simulink model "gm_sampleModel1902_1_sub"  (R2023a)
settings: Solver=VariableStepAuto  StartTime=0.0  StopTime=10.0  RelTol=1e-3
libraries: hdlsllib x2, simulink x1
settings Model: Creator=user1  LastModifiedBy=user1
settings OptimizationCC: BlockReduction=off  ConditionallyExecuteInputs=off
settings DebuggingCC: InheritedTsInSrcMsg=none

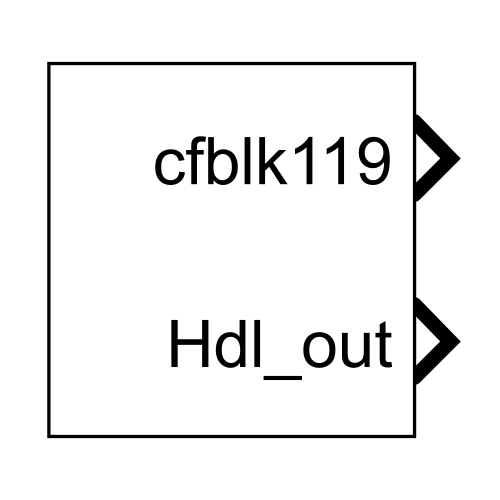
[thumbnail: Simulink's stored preview of the top-level diagram]
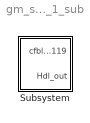
== system gm_sampleModel1902_1_sub ==
  Subsystem : Subsystem

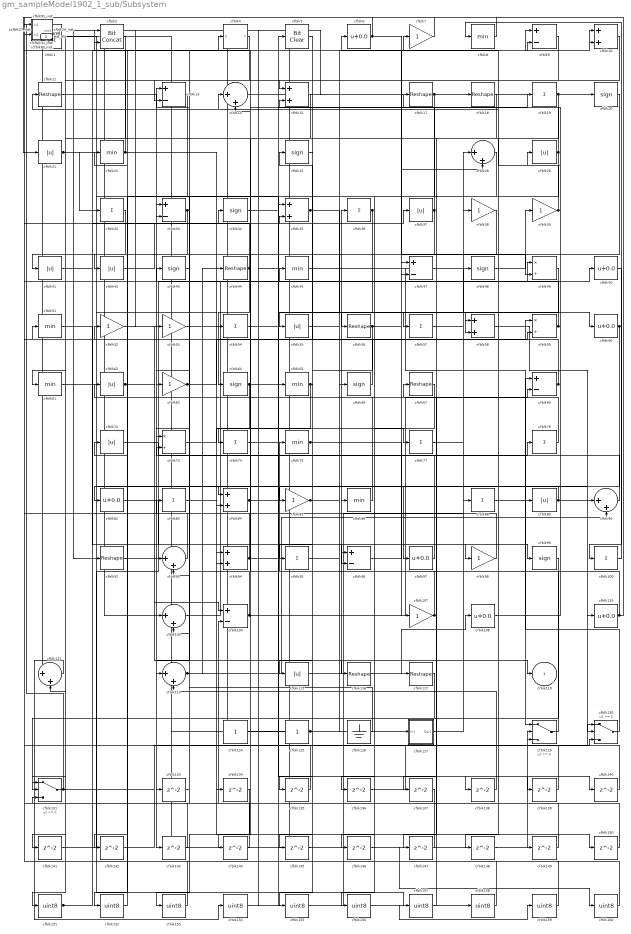
== system gm_sampleModel1902_1_sub/Subsystem ==
  cfblk1 : hdlsllib/Logic and Bit Operations/Interval Test  IntervalClosedRight=on  uplimit=0.5  IntervalClosedLeft=on  lowlimit=-0.5  OutDataTypeStr=uint8
  cfblk{10,15,35,58,84,94} (6 alike) : Sum  OutDataTypeStr=uint8
  cfblk{19,32,36,54,57,74,77,79,83,88,95,100} (12 alike) : Sum  Inputs=+  OutDataTypeStr=uint8
  cfblk{14,28,90,93,103,111,113} (7 alike) : Sum  Inputs=|++  OutDataTypeStr=uint8
  cfblk{9,13,33,47,69,96,104} (7 alike) : Sum  Inputs=+-  OutDataTypeStr=uint8
  cfblk105_inst : Subsystem
  cfblk{7,38..39,52..53,63,85,98,107} (9 alike) : Gain  OutDataTypeStr=uint8
  cfblk{6,50,60,82,97,108,110} (7 alike) : Bias  Bias=0.0  SaturateOnIntegerOverflow=off
  cfblk109_inst : Subsystem
  cfblk{11,17..18,44,56,67,92,116..117} (9 alike) : Reshape
  cfblk112_inst : Subsystem
  cfblk{21,29,37,41..42,55,62,72,89,115} (10 alike) : Abs  OutDataTypeStr=uint8  SaturateOnIntegerOverflow=off
  cfblk124 : Constant  OutDataTypeStr=uint8  SampleTime=-1
  cfblk125 : Constant  OutDataTypeStr=uint8  SampleTime=-1
  cfblk126 : Ground
  cfblk127 : Subsystem
  cfblk129 : Switch  OutDataTypeStr=uint8  SaturateOnIntegerOverflow=off  InputSameDT=off
  cfblk130 : Switch  OutDataTypeStr=uint8  SaturateOnIntegerOverflow=off  InputSameDT=off
  cfblk131 : Switch  OutDataTypeStr=uint8  SaturateOnIntegerOverflow=off  InputSameDT=off
  cfblk{133..150} (18 alike) : Delay  SampleTime=1
  cfblk{151..160} (10 alike) : DataTypeConversion  OutDataTypeStr=uint8  SaturateOnIntegerOverflow=off  RndMeth=Floor
  cfblk2 : hdlsllib/Logic and Bit Operations/Bit Concat  numInputs=2
  cfblk{20,25,34,43,48,64,66,99} (8 alike) : Signum
  cfblk{8,22,45,51,61,65,75,86} (8 alike) : MinMax  OutDataTypeStr=uint8
  cfblk24_inst : Subsystem
  cfblk26_inst : Subsystem
  cfblk27_inst : Subsystem
  cfblk31_inst : Subsystem
  cfblk4 : Subsystem  mask(Detect Rise Nonnegative){vinit=double(0), InputProcessing=Elements as channels (sample based), OutDataTypeStr=uint8}
      mask prompts: vinit "Simulink:masks:InitialCondition_MP"; InputProcessing "Simulink:masks:InputProcessing_MP"; OutDataTypeStr "Simulink:masks:OutputDataType_MP"
      mask help: Simulink:masks:DetectRiseNonnegative_MD
      mask init:
      | InputProcessing = 'Elements as channels (sample based)';
      | OutDataTypeStr = 'uint8';
      | vinit = double(0);
      mask TypeOptions InputProcessing: Simulink:masks:ColumnsAsChannelsFrameBased | Simulink:masks:ElementsAsChannelsSampleBased
      mask TypeOptions OutDataTypeStr: Simulink:masks:uint8 | Simulink:masks:boolean
      mask Display: fprintf('U >= 0\n&  NOT\nU/z >= 0')
  cfblk49 : Product  Inputs=*/  OutDataTypeStr=uint8  RndMeth=Zero  SaturateOnIntegerOverflow=on
  cfblk5 : simulink/Logic and Bit Operations/Bit Clear  iBit=0
      settings: LibrarySourceBlock=|
      | hdlsllib/Logic and Bit
      | Operations/Bit Clear
  cfblk59 : Product  Inputs=*/  OutDataTypeStr=uint8  RndMeth=Zero  SaturateOnIntegerOverflow=on
  cfblk73 : Product  Inputs=*/  OutDataTypeStr=uint8  RndMeth=Zero  SaturateOnIntegerOverflow=on
  cfblk80_inst : Subsystem
  cfblk91_inst : Subsystem
  cfblk119 : Outport  OutDataTypeStr=uint8  SampleTime=1  VectorParamsAs1DForOutWhenUnconnected=off
  Hdl_out : Outport  Port=2  OutDataTypeStr=uint8  SampleTime=1
  wires:
  cfblk1/1 -> cfblk157/1, cfblk111/2
  cfblk10/1 -> cfblk15/1
  cfblk100/1 -> cfblk8/1
  cfblk103/1 -> cfblk45/1
  cfblk104/1 -> cfblk69/2, cfblk112_inst/1(in1)
  cfblk105_inst/1(out1) -> cfblk127/1(In1)
  cfblk107/1 -> cfblk147/1, cfblk36/1
  cfblk108/1 -> cfblk15/2
  cfblk109_inst/1(out1) -> cfblk117/1
  cfblk11/1 -> cfblk143/1
  cfblk110/1 -> cfblk21/1, cfblk75/1
  cfblk111/1 -> cfblk154/1
  cfblk112_inst/1(out1) -> cfblk92/1
  cfblk113/1 -> cfblk90/2, cfblk44/1
  cfblk115/1 -> cfblk86/1
  cfblk116/1 -> cfblk108/1
  cfblk117/1 -> cfblk133/1
  cfblk124/1 -> cfblk35/1
  cfblk125/1 -> cfblk66/1, Hdl_out/1
  cfblk126/1 -> cfblk51/1
  cfblk127/1(Out1) -> cfblk88/1
  cfblk129/1 -> cfblk4/1(U)
  cfblk13/1 -> cfblk152/1
  cfblk130/1 -> cfblk69/1
  cfblk131/1 -> cfblk130/3, cfblk109_inst/2(in2)
  cfblk133/1 -> cfblk103/2
  cfblk134/1 -> cfblk153/1
  cfblk135/1 -> cfblk93/2
  cfblk136/1 -> cfblk130/1
  cfblk137/1 -> cfblk131/3
  cfblk138/1 -> cfblk113/2
  cfblk139/1 -> cfblk91_inst/2(in2)
  cfblk14/1 -> cfblk10/1
  cfblk140/1 -> cfblk105_inst/1(in1)
  cfblk141/1 -> cfblk49/1
  cfblk142/1 -> cfblk129/2
  cfblk143/1 -> cfblk112_inst/2(in2)
  cfblk144/1 -> cfblk27_inst/2(in2)
  cfblk145/1 -> cfblk1/1
  cfblk146/1 -> cfblk160/1
  cfblk147/1 -> cfblk13/1
  cfblk148/1 -> cfblk129/3
  cfblk149/1 -> cfblk104/2
  cfblk15/1 -> cfblk74/1
  cfblk150/1 -> cfblk43/1
  cfblk151/1 -> cfblk35/2, cfblk7/1
  cfblk152/1 -> cfblk2/1
  cfblk153/1 -> cfblk2/2
  cfblk154/1 -> cfblk5/1
  cfblk155/1 -> cfblk38/1
  cfblk156/1 -> cfblk159/1
  cfblk157/1 -> cfblk67/1
  cfblk158/1 -> cfblk52/1
  cfblk159/1 -> cfblk24_inst/1(in1)
  cfblk160/1 -> cfblk24_inst/2(in2)
  cfblk17/1 -> cfblk33/2, cfblk113/1
  cfblk18/1 -> cfblk137/1
  cfblk19/1 -> cfblk148/1, cfblk61/1
  cfblk2/1 -> cfblk151/1
  cfblk20/1 -> cfblk55/1
  cfblk21/1 -> cfblk84/2, cfblk53/1, cfblk32/1, cfblk65/1
  cfblk22/1 -> cfblk80_inst/2(in2), cfblk134/1
  cfblk24_inst/1(out1) -> cfblk158/1
  cfblk25/1 -> cfblk85/1
  cfblk26_inst/1(out1) -> cfblk111/1
  cfblk27_inst/1(out1) -> cfblk103/1
  cfblk28/1 -> cfblk136/1
  cfblk29/1 -> cfblk80_inst/1(in1), cfblk58/2, cfblk33/1
  cfblk31_inst/1(out1) -> cfblk48/1, cfblk18/1
  cfblk32/1 -> cfblk131/2
  cfblk33/1 -> cfblk142/1, cfblk141/1
  cfblk34/1 -> cfblk17/1
  cfblk35/1 -> cfblk58/1, cfblk19/1
  cfblk36/1 -> cfblk42/1, cfblk145/1
  cfblk37/1 -> cfblk26_inst/2(in2), cfblk73/1
  cfblk38/1 -> cfblk146/1
  cfblk39/1 -> cfblk6/1, cfblk11/1
  cfblk4/1(Y) -> cfblk13/2
  cfblk41/1 -> cfblk34/1
  cfblk42/1 -> cfblk37/1
  cfblk43/1 -> cfblk63/1
  cfblk44/1 -> cfblk64/1, cfblk105_inst/2(in2)
  cfblk45/1 -> cfblk129/1
  cfblk47/1 -> cfblk60/1
  cfblk48/1 -> cfblk39/1
  cfblk49/1 -> cfblk95/1
  cfblk5/1 -> cfblk155/1
  cfblk50/1 -> cfblk100/1
  cfblk51/1 -> cfblk99/1
  cfblk52/1 -> cfblk104/1
  cfblk53/1 -> cfblk94/1
  cfblk54/1 -> cfblk56/1
  cfblk55/1 -> cfblk57/1
  cfblk56/1 -> cfblk47/2, cfblk135/1
  cfblk57/1 -> cfblk50/1
  cfblk58/1 -> cfblk130/2
  cfblk59/1 -> cfblk29/1, cfblk26_inst/1(in1)
  cfblk6/1 -> cfblk109_inst/1(in1), cfblk49/2
  cfblk60/1 -> cfblk97/1, cfblk82/1
  cfblk61/1 -> cfblk110/1
  cfblk62/1 -> cfblk96/2, cfblk119/1
  cfblk63/1 -> cfblk59/2, cfblk150/1
  cfblk64/1 -> cfblk94/2, cfblk138/1
  cfblk65/1 -> cfblk115/1, cfblk144/1
  cfblk66/1 -> cfblk25/1
  cfblk67/1 -> cfblk156/1
  cfblk69/1 -> cfblk31_inst/2(in2), cfblk22/1
  cfblk7/1 -> cfblk31_inst/1(in1)
  cfblk72/1 -> cfblk79/1
  cfblk73/1 -> cfblk77/1
  cfblk74/1 -> cfblk96/1
  cfblk75/1 -> cfblk10/2, cfblk107/1
  cfblk77/1 -> cfblk28/1
  cfblk79/1 -> cfblk14/1
  cfblk8/1 -> cfblk27_inst/1(in1)
  cfblk80_inst/1(out1) -> cfblk54/1
  cfblk82/1 -> cfblk98/1
  cfblk83/1 -> cfblk116/1
  cfblk84/1 -> cfblk47/1, cfblk140/1
  cfblk85/1 -> cfblk9/2, cfblk59/1
  cfblk86/1 -> cfblk62/1
  cfblk88/1 -> cfblk89/1
  cfblk89/1 -> cfblk90/1, cfblk84/1
  cfblk9/1 -> cfblk41/1
  cfblk90/1 -> cfblk73/2
  cfblk91_inst/1(out1) -> cfblk20/1, cfblk149/1
  cfblk92/1 -> cfblk93/1
  cfblk93/1 -> cfblk91_inst/1(in1)
  cfblk94/1 -> cfblk72/1, cfblk139/1
  cfblk95/1 -> cfblk9/1
  cfblk96/1 -> cfblk28/2
  cfblk97/1 -> cfblk14/2
  cfblk98/1 -> cfblk83/1
  cfblk99/1 -> cfblk131/1

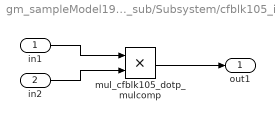
== system gm_sampleModel1902_1_sub/Subsystem/cfblk105_inst ==
  in1 : Inport  OutDataTypeStr=uint8  SampleTime=1
  in2 : Inport  Port=2  OutDataTypeStr=uint8  SampleTime=1
  mul_cfblk105_dotp_mulcomp : Product  Inputs=**  OutDataTypeStr=uint8  SampleTime=1
  out1 : Outport  OutDataTypeStr=uint8  SampleTime=1
  wires:
  in1/1 -> mul_cfblk105_dotp_mulcomp/1
  in2/1 -> mul_cfblk105_dotp_mulcomp/2
  mul_cfblk105_dotp_mulcomp/1 -> out1/1

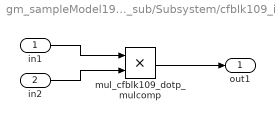
== system gm_sampleModel1902_1_sub/Subsystem/cfblk109_inst ==
  in1 : Inport  OutDataTypeStr=uint8  SampleTime=1
  in2 : Inport  Port=2  OutDataTypeStr=uint8  SampleTime=1
  mul_cfblk109_dotp_mulcomp : Product  Inputs=**  OutDataTypeStr=uint8  SampleTime=1
  out1 : Outport  OutDataTypeStr=uint8  SampleTime=1
  wires:
  in1/1 -> mul_cfblk109_dotp_mulcomp/1
  in2/1 -> mul_cfblk109_dotp_mulcomp/2
  mul_cfblk109_dotp_mulcomp/1 -> out1/1

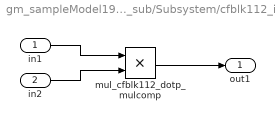
== system gm_sampleModel1902_1_sub/Subsystem/cfblk112_inst ==
  in1 : Inport  OutDataTypeStr=uint8  SampleTime=1
  in2 : Inport  Port=2  OutDataTypeStr=uint8  SampleTime=1
  mul_cfblk112_dotp_mulcomp : Product  Inputs=**  OutDataTypeStr=uint8  SampleTime=1
  out1 : Outport  OutDataTypeStr=uint8  SampleTime=1
  wires:
  in1/1 -> mul_cfblk112_dotp_mulcomp/1
  in2/1 -> mul_cfblk112_dotp_mulcomp/2
  mul_cfblk112_dotp_mulcomp/1 -> out1/1

== system gm_sampleModel1902_1_sub/Subsystem/cfblk127 ==
  In1 : Inport  OutDataTypeStr=uint8  PortDimensions=1  SampleTime=1
  Out1 : Outport  SampleTime=1
  wires:
  In1/1 -> Out1/1

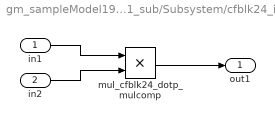
== system gm_sampleModel1902_1_sub/Subsystem/cfblk24_inst ==
  in1 : Inport  OutDataTypeStr=uint8  SampleTime=1
  in2 : Inport  Port=2  OutDataTypeStr=uint8  SampleTime=1
  mul_cfblk24_dotp_mulcomp : Product  Inputs=**  OutDataTypeStr=uint8  SampleTime=1
  out1 : Outport  OutDataTypeStr=uint8  SampleTime=1
  wires:
  in1/1 -> mul_cfblk24_dotp_mulcomp/1
  in2/1 -> mul_cfblk24_dotp_mulcomp/2
  mul_cfblk24_dotp_mulcomp/1 -> out1/1

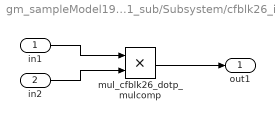
== system gm_sampleModel1902_1_sub/Subsystem/cfblk26_inst ==
  in1 : Inport  OutDataTypeStr=uint8  SampleTime=1
  in2 : Inport  Port=2  OutDataTypeStr=uint8  SampleTime=1
  mul_cfblk26_dotp_mulcomp : Product  Inputs=**  OutDataTypeStr=uint8  SampleTime=1
  out1 : Outport  OutDataTypeStr=uint8  SampleTime=1
  wires:
  in1/1 -> mul_cfblk26_dotp_mulcomp/1
  in2/1 -> mul_cfblk26_dotp_mulcomp/2
  mul_cfblk26_dotp_mulcomp/1 -> out1/1

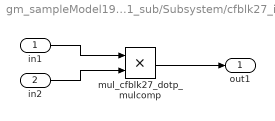
== system gm_sampleModel1902_1_sub/Subsystem/cfblk27_inst ==
  in1 : Inport  OutDataTypeStr=uint8  SampleTime=1
  in2 : Inport  Port=2  OutDataTypeStr=uint8  SampleTime=1
  mul_cfblk27_dotp_mulcomp : Product  Inputs=**  OutDataTypeStr=uint8  SampleTime=1
  out1 : Outport  OutDataTypeStr=uint8  SampleTime=1
  wires:
  in1/1 -> mul_cfblk27_dotp_mulcomp/1
  in2/1 -> mul_cfblk27_dotp_mulcomp/2
  mul_cfblk27_dotp_mulcomp/1 -> out1/1

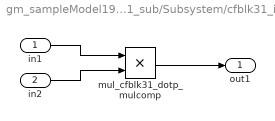
== system gm_sampleModel1902_1_sub/Subsystem/cfblk31_inst ==
  in1 : Inport  OutDataTypeStr=uint8  SampleTime=1
  in2 : Inport  Port=2  OutDataTypeStr=uint8  SampleTime=1
  mul_cfblk31_dotp_mulcomp : Product  Inputs=**  OutDataTypeStr=uint8  SampleTime=1
  out1 : Outport  OutDataTypeStr=uint8  SampleTime=1
  wires:
  in1/1 -> mul_cfblk31_dotp_mulcomp/1
  in2/1 -> mul_cfblk31_dotp_mulcomp/2
  mul_cfblk31_dotp_mulcomp/1 -> out1/1

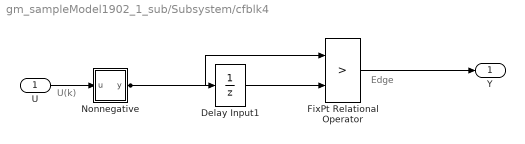
== system gm_sampleModel1902_1_sub/Subsystem/cfblk4 ==
  note: U(k)
  note: Edge
  U : Inport  OutDataTypeStr=uint8  SampleTime=1
  Delay Input1 : UnitDelay  Description=Store in Global RAM  DisableCoverage=on  InitialCondition=vinit  SampleTime=-1  HasFrameUpgradeWarning=on
  FixPt Relational Operator : RelationalOperator  Operator=>  OutDataTypeStr=fixdt(0, 8)  ZeroCross=off  InputSameDT=off
  Nonnegative : Subsystem  mask(Compare To Zero){relop=>=, OutDataTypeStr=boolean, ZeroCross=off}
      mask prompts: relop "Simulink:masks:Operator_MP"; OutDataTypeStr "Simulink:masks:OutputDataType_MP"; ZeroCross "Simulink:masks:EnableZerocrossingDetection_MP"
      mask help: Simulink:masks:CompareToZero_MD
      mask init:
      | OutDataTypeStr = 'boolean';
      | ZeroCross = 'off';
      | blkName = 'sampleModel1902_1_sub/Subsystem/cfblk4/Nonnegative';
      | relop = '>=';
      | setValue = 'boolean';
      mask TypeOptions relop: == | ~= | < | <= | >= | >
      mask TypeOptions OutDataTypeStr: Simulink:masks:uint8 | Simulink:masks:boolean
      mask Callback ZeroCross: sl('zeroCrossEnable', gcbh);
      mask Display: disp([relop,' 0'])
  Y : Outport  SampleTime=1
  wires:
  U/1 -> Nonnegative/1(u)
  Delay Input1/1 -> FixPt Relational Operator/2
  FixPt Relational Operator/1 -> Y/1
  Nonnegative/1(y) -> FixPt Relational Operator/1, Delay Input1/1

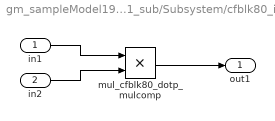
== system gm_sampleModel1902_1_sub/Subsystem/cfblk80_inst ==
  in1 : Inport  OutDataTypeStr=uint8  SampleTime=1
  in2 : Inport  Port=2  OutDataTypeStr=uint8  SampleTime=1
  mul_cfblk80_dotp_mulcomp : Product  Inputs=**  OutDataTypeStr=uint8  SampleTime=1
  out1 : Outport  OutDataTypeStr=uint8  SampleTime=1
  wires:
  in1/1 -> mul_cfblk80_dotp_mulcomp/1
  in2/1 -> mul_cfblk80_dotp_mulcomp/2
  mul_cfblk80_dotp_mulcomp/1 -> out1/1

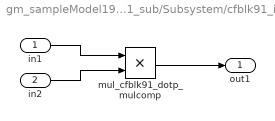
== system gm_sampleModel1902_1_sub/Subsystem/cfblk91_inst ==
  in1 : Inport  OutDataTypeStr=uint8  SampleTime=1
  in2 : Inport  Port=2  OutDataTypeStr=uint8  SampleTime=1
  mul_cfblk91_dotp_mulcomp : Product  Inputs=**  OutDataTypeStr=uint8  SampleTime=1
  out1 : Outport  OutDataTypeStr=uint8  SampleTime=1
  wires:
  in1/1 -> mul_cfblk91_dotp_mulcomp/1
  in2/1 -> mul_cfblk91_dotp_mulcomp/2
  mul_cfblk91_dotp_mulcomp/1 -> out1/1

== system gm_sampleModel1902_1_sub/Subsystem/cfblk4/Nonnegative ==
  u : Inport  OutDataTypeStr=uint8  SampleTime=1
  Compare : RelationalOperator  OutDataTypeStr=boolean  ZeroCross=off
  Constant : Constant  DisableCoverage=on  Value=0  OutDataTypeStr=Inherit: Inherit via back propagation  SampleTime=-1  PreserveConstantTs=on
  y : Outport  SampleTime=1
  wires:
  u/1 -> Compare/1
  Compare/1 -> y/1
  Constant/1 -> Compare/2
